simulink model "QBot2e_Image_Proc_Blob_Tracking"  (Simulink 8.9)
settings: Solver=ode1  StartTime=0.0  StopTime=inf  FixedStep=0.01  RelTol=1e-3  EnableMultiTasking=on
undefined symbols (not defined in the file): gcbh, HIL, JPEG, qc_get_step_size, Video3D, video_display_show
libraries: quarc_library x14
settings Model: Creator=drmadill  LastModifiedBy=User  SimulationMode=external  ExtModeTrigDuration=2
settings SolverCC: PositivePriorityOrder=on
settings OptimizationCC: ExpressionDepthLimit=2147483647  LifeSpan=auto
settings DebuggingCC: SolverPrmCheckMsg=warning
settings RTWCC: SystemTargetFile=quarc_linux_pi_3.tlc  TemplateMakefile=quarc_linux_pi_3_tmf  Description=QUARC Linux Raspberry Pi 3 Target
settings STFCustomTargetCC: TargetLibSuffix=.a  TargetPreCompLibLocation=C:\PROGRA~3\QUARC\lib\2019b\LINUX_~1\release  ConcurrentExecutionCompliant=on  SystemTargetFile=quarc_linux_pi_3.tlc
settings GRTTargetCC: TargetLibSuffix=.a  TargetPreCompLibLocation=C:\PROGRA~3\QUARC\lib\2017a\LICFC8~1\release  ParMdlRefBuildCompliant=off  CompOptLevelCompliant=off  GeneratePreprocessorConditionals=Use local settings  MatFileLogging=off  CPPClassGenCompliant=off  UseToolchainInfoCompliant=off  ExtMode=on  ExtModeMexFile=quarc_comm  ExtModeMexArgs='-w -d /tmp -uri %u'
settings ConfigComp: CovSFcnEnable=off

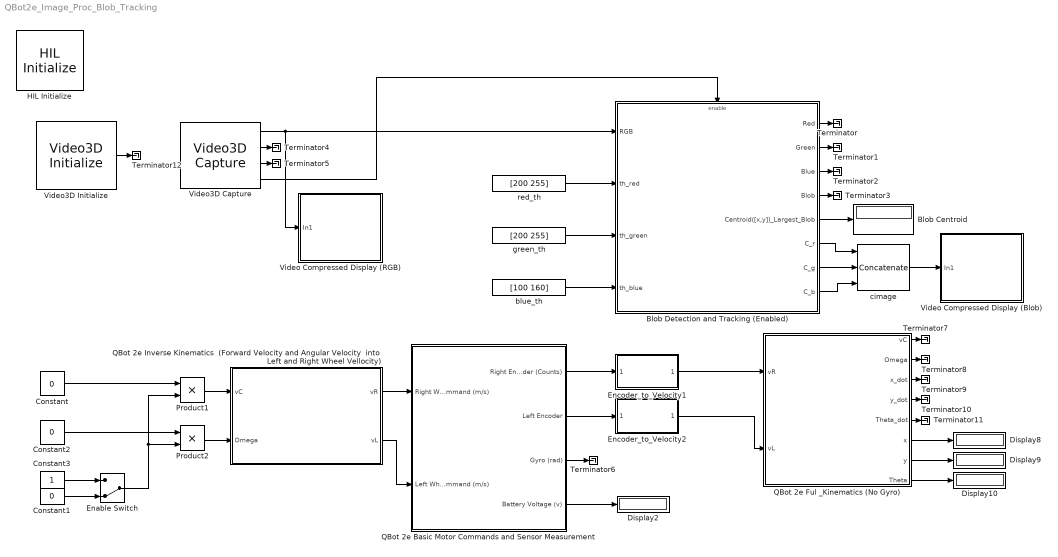
== system QBot2e_Image_Proc_Blob_Tracking ==
  " Blob Detection and Tracking (Enabled)" : Subsystem  TreatAsAtomicUnit=on
  Blob Centroid : Display
  Constant : Constant  Value=0
  Constant1 : Constant  Value=0
  Constant2 : Constant  Value=0
  Constant3 : Constant
  Display{2,8..10} (4 alike) : Display
  Enable Switch : ManualSwitch  CurrentSetting=0
  Encoder_to_Velocity1 : Subsystem
  Encoder_to_Velocity2 : Subsystem
  HIL Initialize : quarc_library/Data Acquisition/Generic/Configuration/HIL Initialize  Priority=-99  object_name=HIL-1  board_type=qbot2e  board_number=0  board_options=pwm0_en=1;pwm0_pin=12;pwm1_en=1;pwm1_pin=13;  exclusive=off  active=off  hardware_clocks=[]  clock_modes=[]  initial_clock_frequencies=[]  set_clock_params_at_start=off  set_clock_params_at_switch_in=off  set_clock_frequencies_at_start=off  set_clock_frequencies_at_switch_in=off  analog_input_channels=[0:5]  analog_input_configurations=[]  analog_input_maximums=[16.5 3.3 3.3 3.3 3.3 3.3]  analog_input_minimums=[0 0 0 0 0 0]  set_analog_input_params_at_start=off  set_analog_input_params_at_switch_in=off  analog_output_channels=[]  analog_output_maximums=[]  analog_output_minimums=[]  initial_analog_outputs=[]  final_analog_outputs=[]  watchdog_analog_outputs=[]  set_analog_output_params_at_start=off  set_analog_output_params_at_switch_in=off  set_analog_outputs_at_start=off  set_analog_outputs_at_switch_in=off  set_analog_outputs_at_terminate=off  set_analog_outputs_at_switch_out=off  set_analog_outputs_on_watchdog=off  digital_input_channels=[28:58]  digital_output_channels=[28:31]  digital_output_configuration=[]  initial_digital_outputs=[0]  final_digital_outputs=[0]  watchdog_digital_outputs=[]  set_digital_output_params_at_start=off  set_digital_output_params_at_switch_in=off  set_digital_outputs_at_start=on  set_digital_outputs_at_switch_in=off  set_digital_outputs_at_terminate=on  set_digital_outputs_at_switch_out=off  set_digital_outputs_on_watchdog=off  encoder_channels=[0:1]  quadrature=[4]  encoder_filter_frequency=[]  initial_encoder_counts=[0]  set_encoder_params_at_start=on  set_encoder_params_at_switch_in=off  set_encoder_counts_at_start=on  set_encoder_counts_at_switch_in=off  pwm_channels=[0:1]  pwm_modes=0  pwm_frequency=100e6 / 4095  pwm_configuration=[0]  pwm_alignment=[0]  pwm_polarity=[1]  pwm_leading_deadband=[]  pwm_trailing_deadband=[]  initial_pwm_outputs=[0]  final_pwm_outputs=[0]  watchdog_pwm_outputs=[]  set_pwm_params_at_start=on  set_pwm_params_at_switch_in=off  set_pwm_outputs_at_start=on  set_pwm_outputs_at_switch_in=off  set_pwm_outputs_at_terminate=on  set_pwm_outputs_at_switch_out=off  set_pwm_outputs_on_watchdog=off  other_output_channels=[2000:2001 14000 16000]  initial_other_outputs=[0 0 0 7]  final_other_outputs=[0 0 0 7]  watchdog_other_outputs=[]  set_other_outputs_at_start=on  set_other_outputs_at_switch_in=off  set_other_outputs_at_terminate=on  set_other_outputs_at_switch_out=off  set_other_outputs_on_watchdog=off
  Product1 : Product  RndMeth=Zero
  Product2 : Product  RndMeth=Zero
  QBot 2e Basic Motor Commands and Sensor Measurement : Subsystem
  QBot 2e Ful _Kinematics (No Gyro) : Subsystem
  QBot 2e Inverse Kinematics  (Forward Velocity and Angular Velocity  into Left and Right Wheel Vellocity) : Subsystem
  Terminator{,1..12} (13 alike) : Terminator
  Video Compressed Display (Blob) : Subsystem  LoadFcn=set_param(gcbh, 'UserData', gcb);  StartFcn=video_display_show([gcb, '/Video Display'], 'add', gcb);  mask(Video Compressed Display){algorithm=JPEG, quality=50, sample_time=-1, use_hardware=on}
      mask prompts: algorithm "Compression algorithm:"; quality "Compression quality (0-100):"; sample_time "Sample time (seconds):"; use_hardware "Use hardware acceleration for video display"
      mask help: Displays a video stream on the host, using compression to minimize bandwidth.
      mask init:
      | qc_set_display('Video\nCompressed\nDisplay');
      settings: UndoDeleteFcn=set_param(gcbh, 'UserData', gcb);  OpenFcn=video_display_show([gcb, '/Video Display'], 'show', gcb);  PreDeleteFcn=video_display_show([gcb, '/Video Display'], 'delete');
      settings: CopyFcn=|
      | set_param(gcbh, 'UserData', gcb);
      | set_param(gcbh, 'LinkStatus', 'none');
      settings: NameChangeFcn=|
      | video_display_show([get_param(gcbh, 'UserData'), '/Video Display'], 'rename', [gcb, '/Video Display']);
      | video_display_show([gcb, '/Video Display'], 'add', gcb);
      | set_param(gcbh, 'UserData', gcb);
      mask Help: web(qc_get_block_help_path(gcb));
      mask TypeOptions algorithm: Image Compress/algorithm
      mask TypeOptions quality: Image Compress/quality
      mask TypeOptions sample_time: Video Display/sample_time
      mask TypeOptions use_hardware: Video Display/use_hardware
      mask Display:
      | patch([0.98591 0.98591 0.62618 0.59072 0.56147   0.536   0.536  0.5441 0.56912 0.59207 0.60881 0.62276 0.63527 0.64364  0.6485  0.6485 0.64706 0.64499 0.63662 0.62411 0.61232 0.59837 0.58307 0.56147   0.536   0.536  0.5441  0.5747 0.60953 0.63662 0.67001  0.7034 0.72851 0.75425 0.77927 0.80294 0.82454 0.84119 0.85865 0.87395 0.88574 0.89339  0.8969 0.89969 0.89969 0.89267  0.8816 0.87044 0.85649  0.8384 0.81824 0.80294 0.78764 0.77513 0.76676 0.75776 0.76397 0.77513 0.79178 0.80987 0.82796 0.84326 0.86207 0.98528],[0.18689 0.05522 0.05522 0.05171 0.05171    0.05 0.18338 0.18338 0.19148 0.20435 0.22298 0.24863 0.28589 0.33125 0.38138 0.55139 0.59801 0.63761 0.68189 0.72149 0.74939 0.76694 0.77855 0.79367 0.79952 0.92768 0.92768 0.92768 0.92417 0.92066 0.91364  0.9032 0.89384 0.88106 0.86594 0.85073 0.82634 0.80537 0.77855 0.74363 0.70403 0.65858 0.61079 0.59099 0.41513 0.37202 0.31847 0.29048 0.25556 0.23342  0.2102 0.19382 0.18221 0.17285 0.16943 0.16124  0.1589 0.16241 0.16709 0.17168  0.1787 0.18221 0.18689 0.18689],[0.9,0.90,0.91])
      | patch([0.536 0.52601 0.46823 0.44528 0.41603 0.39101 0.35555 0.33116 0.31451 0.29291  0.2804 0.26717 0.25322 0.23999 0.22406 0.20732 0.19337 0.17528 0.15935 0.14396 0.13217 0.11759 0.10922 0.10085 0.09671 0.09392 0.09041 0.08906 0.08906 0.09464  0.0995 0.10778 0.11894 0.13145 0.14675 0.16349 0.17672 0.19409 0.20732 0.22406 0.23999 0.26159 0.27833 0.29849 0.31793 0.33602 0.35411 0.37085 0.39245 0.41603   0.536   0.536 0.53159 0.46409   0.446 0.42026 0.39587 0.37571 0.36113 0.34925 0.34088 0.33809 0.33809 0.34088 0.34583 0.35627 0.36392 0.38129 0.39587 0.41117 0.42719 0.44672  0.4676 0.48353 0.48353 0.52394   0.536],[0.05 0.04829 0.04712 0.04712 0.04829 0.05063 0.05405 0.05873 0.06107 0.06692 0.07043 0.07619 0.08087 0.08672 0.09482 0.10652 0.11696 0.13325  0.1508 0.17168 0.19499 0.22415 0.25439 0.28472 0.31379 0.35456 0.38489 0.41513 0.58055 0.63878 0.68774 0.72149 0.75641 0.78089 0.80537 0.82859 0.84029 0.85658 0.86594 0.87404  0.8834 0.89267 0.90086 0.90788 0.91247 0.91832 0.92066   0.923 0.92651 0.92768 0.92768 0.79952 0.79952 0.79952 0.79718 0.78899 0.77153 0.75056 0.72149 0.68072 0.62249  0.5549 0.41396 0.37085 0.33242 0.28121 0.25205 0.22181 0.20552 0.19499 0.18572 0.18221 0.17753 0.17636 0.17753  0.1787  0.1787],[0.9,0.90,0.91])
      | disp('Video\nCompressed\nDisplay');
  Video Compressed Display (RGB) : Subsystem  LoadFcn=set_param(gcbh, 'UserData', gcb);  StartFcn=video_display_show([gcb, '/Video Display'], 'add', gcb);  mask(Video Compressed Display){algorithm=JPEG, quality=50, sample_time=-1, use_hardware=on}
      mask prompts: algorithm "Compression algorithm:"; quality "Compression quality (0-100):"; sample_time "Sample time (seconds):"; use_hardware "Use hardware acceleration for video display"
      mask help: Displays a video stream on the host, using compression to minimize bandwidth.
      mask init:
      | qc_set_display('Video\nCompressed\nDisplay');
      settings: UndoDeleteFcn=set_param(gcbh, 'UserData', gcb);  OpenFcn=video_display_show([gcb, '/Video Display'], 'show', gcb);  PreDeleteFcn=video_display_show([gcb, '/Video Display'], 'delete');
      settings: CopyFcn=|
      | set_param(gcbh, 'UserData', gcb);
      | set_param(gcbh, 'LinkStatus', 'none');
      settings: NameChangeFcn=|
      | video_display_show([get_param(gcbh, 'UserData'), '/Video Display'], 'rename', [gcb, '/Video Display']);
      | video_display_show([gcb, '/Video Display'], 'add', gcb);
      | set_param(gcbh, 'UserData', gcb);
      mask Help: web(qc_get_block_help_path(gcb));
      mask TypeOptions algorithm: Image Compress/algorithm
      mask TypeOptions quality: Image Compress/quality
      mask TypeOptions sample_time: Video Display/sample_time
      mask TypeOptions use_hardware: Video Display/use_hardware
      mask Display:
      | patch([0.98591 0.98591 0.62618 0.59072 0.56147   0.536   0.536  0.5441 0.56912 0.59207 0.60881 0.62276 0.63527 0.64364  0.6485  0.6485 0.64706 0.64499 0.63662 0.62411 0.61232 0.59837 0.58307 0.56147   0.536   0.536  0.5441  0.5747 0.60953 0.63662 0.67001  0.7034 0.72851 0.75425 0.77927 0.80294 0.82454 0.84119 0.85865 0.87395 0.88574 0.89339  0.8969 0.89969 0.89969 0.89267  0.8816 0.87044 0.85649  0.8384 0.81824 0.80294 0.78764 0.77513 0.76676 0.75776 0.76397 0.77513 0.79178 0.80987 0.82796 0.84326 0.86207 0.98528],[0.18689 0.05522 0.05522 0.05171 0.05171    0.05 0.18338 0.18338 0.19148 0.20435 0.22298 0.24863 0.28589 0.33125 0.38138 0.55139 0.59801 0.63761 0.68189 0.72149 0.74939 0.76694 0.77855 0.79367 0.79952 0.92768 0.92768 0.92768 0.92417 0.92066 0.91364  0.9032 0.89384 0.88106 0.86594 0.85073 0.82634 0.80537 0.77855 0.74363 0.70403 0.65858 0.61079 0.59099 0.41513 0.37202 0.31847 0.29048 0.25556 0.23342  0.2102 0.19382 0.18221 0.17285 0.16943 0.16124  0.1589 0.16241 0.16709 0.17168  0.1787 0.18221 0.18689 0.18689],[0.9,0.90,0.91])
      | patch([0.536 0.52601 0.46823 0.44528 0.41603 0.39101 0.35555 0.33116 0.31451 0.29291  0.2804 0.26717 0.25322 0.23999 0.22406 0.20732 0.19337 0.17528 0.15935 0.14396 0.13217 0.11759 0.10922 0.10085 0.09671 0.09392 0.09041 0.08906 0.08906 0.09464  0.0995 0.10778 0.11894 0.13145 0.14675 0.16349 0.17672 0.19409 0.20732 0.22406 0.23999 0.26159 0.27833 0.29849 0.31793 0.33602 0.35411 0.37085 0.39245 0.41603   0.536   0.536 0.53159 0.46409   0.446 0.42026 0.39587 0.37571 0.36113 0.34925 0.34088 0.33809 0.33809 0.34088 0.34583 0.35627 0.36392 0.38129 0.39587 0.41117 0.42719 0.44672  0.4676 0.48353 0.48353 0.52394   0.536],[0.05 0.04829 0.04712 0.04712 0.04829 0.05063 0.05405 0.05873 0.06107 0.06692 0.07043 0.07619 0.08087 0.08672 0.09482 0.10652 0.11696 0.13325  0.1508 0.17168 0.19499 0.22415 0.25439 0.28472 0.31379 0.35456 0.38489 0.41513 0.58055 0.63878 0.68774 0.72149 0.75641 0.78089 0.80537 0.82859 0.84029 0.85658 0.86594 0.87404  0.8834 0.89267 0.90086 0.90788 0.91247 0.91832 0.92066   0.923 0.92651 0.92768 0.92768 0.79952 0.79952 0.79952 0.79718 0.78899 0.77153 0.75056 0.72149 0.68072 0.62249  0.5549 0.41396 0.37085 0.33242 0.28121 0.25205 0.22181 0.20552 0.19499 0.18572 0.18221 0.17753 0.17636 0.17753  0.1787  0.1787],[0.9,0.90,0.91])
      | disp('Video\nCompressed\nDisplay');
  Video3D Capture : quarc_library/Multimedia/Video3D Capture  object_name=Video3D-1  stream_type=RGB  stream_index=0  resolution=640 x 480  width=640  height=480  output_format=MATLAB RGB (HxWx3)  data_type=uint8  sample_time=qc_get_step_size * ceil(0.033 / qc_get_step_size)  brightness_override=off  brightness=50.0  contrast_override=off  contrast=50.0  hue_override=off  hue=50.0  saturation_override=off  saturation=50.0  sharpness_override=off  sharpness=50.0  gamma_override=off  gamma=50.0  gain_override=off  gain=50.0  backlightcompensation_override=off  backlightcompensation=50.0  whitebalance_override=Automatic white balance  whitebalance=50.0  exposure_override=Automatic exposure  exposure=30.0  emitter=Enable laser emitter  preset=Do not set camera presets
  Video3D Initialize : quarc_library/Multimedia/Video3D Initialize  object_name=Video3D-1  source=Device  identifier=0  file=sample.bag  sample_time=qc_get_step_size * ceil(0.033 / qc_get_step_size)  active=on
  blue_th : Constant  Value=[100 160]
  cimage : Concatenate  NumInputs=3  Mode=Multidimensional array  ConcatenateDimension=3
  green_th : Constant  Value=[200 255]
  red_th : Constant  Value=[200 255]
  wires:
  red_th/1 -> " Blob Detection and Tracking (Enabled)"/2(th_red)
  green_th/1 -> " Blob Detection and Tracking (Enabled)"/3(th_green)
  blue_th/1 -> " Blob Detection and Tracking (Enabled)"/4(th_blue)
  " Blob Detection and Tracking (Enabled)"/5(Centroid([x,y])_Largest_Blob) -> Blob Centroid/1
  " Blob Detection and Tracking (Enabled)"/6(C_r) -> cimage/1
  " Blob Detection and Tracking (Enabled)"/7(C_g) -> cimage/2
  " Blob Detection and Tracking (Enabled)"/8(C_b) -> cimage/3
  Constant3/1 -> Enable Switch/1
  Constant1/1 -> Enable Switch/2
  QBot 2e Basic Motor Commands and Sensor Measurement/1(Right Encoder (Counts)) -> Encoder_to_Velocity1/1(Encoder)
  QBot 2e Ful _Kinematics (No Gyro)/8(Theta) -> Display10/1
  QBot 2e Ful _Kinematics (No Gyro)/7(y) -> Display9/1
  QBot 2e Ful _Kinematics (No Gyro)/6(x) -> Display8/1
  Encoder_to_Velocity1/1(Velocity) -> QBot 2e Ful _Kinematics (No Gyro)/1(vR)
  Encoder_to_Velocity2/1(Velocity) -> QBot 2e Ful _Kinematics (No Gyro)/2(vL)
  Constant/1 -> Product1/1
  Constant2/1 -> Product2/1
  QBot 2e Inverse Kinematics  (Forward Velocity and Angular Velocity  into Left and Right Wheel Vellocity)/1(vR) -> QBot 2e Basic Motor Commands and Sensor Measurement/1(Right Wheel Command (m/s))
  QBot 2e Inverse Kinematics  (Forward Velocity and Angular Velocity  into Left and Right Wheel Vellocity)/2(vL) -> QBot 2e Basic Motor Commands and Sensor Measurement/2(Left Wheel Command (m/s))
  Product1/1 -> QBot 2e Inverse Kinematics  (Forward Velocity and Angular Velocity  into Left and Right Wheel Vellocity)/1(vC)
  Product2/1 -> QBot 2e Inverse Kinematics  (Forward Velocity and Angular Velocity  into Left and Right Wheel Vellocity)/2(Omega)
  Enable Switch/1 -> Product1/2, Product2/2
  " Blob Detection and Tracking (Enabled)"/1(Red) -> Terminator/1
  " Blob Detection and Tracking (Enabled)"/2(Green) -> Terminator1/1
  " Blob Detection and Tracking (Enabled)"/3(Blue) -> Terminator2/1
  " Blob Detection and Tracking (Enabled)"/4(Blob) -> Terminator3/1
  QBot 2e Ful _Kinematics (No Gyro)/1(vC) -> Terminator7/1
  QBot 2e Ful _Kinematics (No Gyro)/2(Omega) -> Terminator8/1
  QBot 2e Ful _Kinematics (No Gyro)/3(x_dot) -> Terminator9/1
  QBot 2e Ful _Kinematics (No Gyro)/4(y_dot) -> Terminator10/1
  QBot 2e Ful _Kinematics (No Gyro)/5(Theta_dot) -> Terminator11/1
  cimage/1 -> Video Compressed Display (Blob)/1(In1)
  QBot 2e Basic Motor Commands and Sensor Measurement/2(Left Encoder) -> Encoder_to_Velocity2/1(Encoder)
  QBot 2e Basic Motor Commands and Sensor Measurement/4(Battery Voltage (v)) -> Display2/1
  QBot 2e Basic Motor Commands and Sensor Measurement/3(Gyro (rad)) -> Terminator6/1
  Video3D Initialize/1 -> Terminator12/1
  Video3D Capture/4 -> " Blob Detection and Tracking (Enabled)"/Enable
  Video3D Capture/1 -> Video Compressed Display (RGB)/1(In1), " Blob Detection and Tracking (Enabled)"/1(RGB)
  Video3D Capture/2 -> Terminator4/1
  Video3D Capture/3 -> Terminator5/1

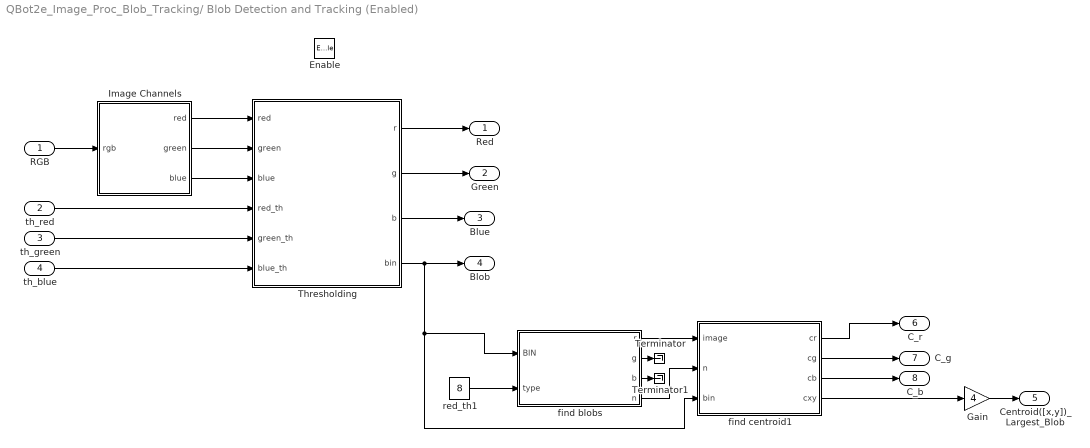
== system QBot2e_Image_Proc_Blob_Tracking/ Blob Detection and Tracking (Enabled) ==
  RGB : Inport
  th_red : Inport  Port=2
  th_green : Inport  Port=3
  th_blue : Inport  Port=4
  Enable : EnablePort
  Gain : Gain  Gain=4
  Image Channels : Subsystem
  Terminator : Terminator
  Terminator1 : Terminator
  Thresholding : MATLAB Function  TreatAsAtomicUnit=on
  find blobs : MATLAB Function  TreatAsAtomicUnit=on
  find centroid1 : MATLAB Function  TreatAsAtomicUnit=on
  red_th1 : Constant  Value=8
  Red : Outport
  Green : Outport  Port=2
  Blue : Outport  Port=3
  Blob : Outport  Port=4
  Centroid([x,y])_Largest_Blob : Outport  Port=5
  C_r : Outport  Port=6
  C_g : Outport  Port=7
  C_b : Outport  Port=8
  wires:
  th_red/1 -> Thresholding/4(red_th)
  th_green/1 -> Thresholding/5(green_th)
  th_blue/1 -> Thresholding/6(blue_th)
  Thresholding/1(r) -> Red/1
  Thresholding/2(g) -> Green/1
  Thresholding/3(b) -> Blue/1
  red_th1/1 -> find blobs/2(type)
  find blobs/1(r) -> find centroid1/1(image)
  find blobs/4(n) -> find centroid1/2(n)
  Gain/1 -> Centroid([x,y])_Largest_Blob/1
  Thresholding/4(bin) -> Blob/1, find blobs/1(BIN), find centroid1/3(bin)
  find centroid1/4(cxy) -> Gain/1
  find centroid1/1(cr) -> C_r/1
  find centroid1/2(cg) -> C_g/1
  find centroid1/3(cb) -> C_b/1
  Image Channels/1(red) -> Thresholding/1(red)
  Image Channels/2(green) -> Thresholding/2(green)
  Image Channels/3(blue) -> Thresholding/3(blue)
  RGB/1 -> Image Channels/1(rgb)
  find blobs/2(g) -> Terminator/1
  find blobs/3(b) -> Terminator1/1

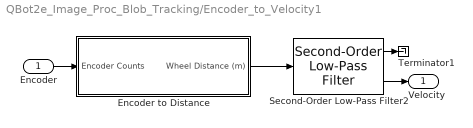
== system QBot2e_Image_Proc_Blob_Tracking/Encoder_to_Velocity1 ==
  Encoder : Inport
  Encoder to Distance : Subsystem
  Second-Order Low-Pass Filter2 : quarc_library/Continuous/Second-Order Low-Pass Filter  params_source=Internal (dialog parameters)  input_width=10  input_zeta=1  input_init=0
  Terminator1 : Terminator
  Velocity : Outport
  wires:
  Second-Order Low-Pass Filter2/1 -> Terminator1/1
  Encoder to Distance/1(Wheel Distance (m)) -> Second-Order Low-Pass Filter2/1
  Encoder/1 -> Encoder to Distance/1(Encoder Counts)
  Second-Order Low-Pass Filter2/2 -> Velocity/1

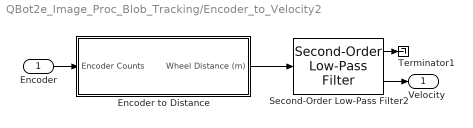
== system QBot2e_Image_Proc_Blob_Tracking/Encoder_to_Velocity2 ==
  Encoder : Inport
  Encoder to Distance : Subsystem
  Second-Order Low-Pass Filter2 : quarc_library/Continuous/Second-Order Low-Pass Filter  params_source=Internal (dialog parameters)  input_width=10  input_zeta=1  input_init=0
  Terminator1 : Terminator
  Velocity : Outport
  wires:
  Second-Order Low-Pass Filter2/2 -> Velocity/1
  Encoder/1 -> Encoder to Distance/1(Encoder Counts)
  Encoder to Distance/1(Wheel Distance (m)) -> Second-Order Low-Pass Filter2/1
  Second-Order Low-Pass Filter2/1 -> Terminator1/1

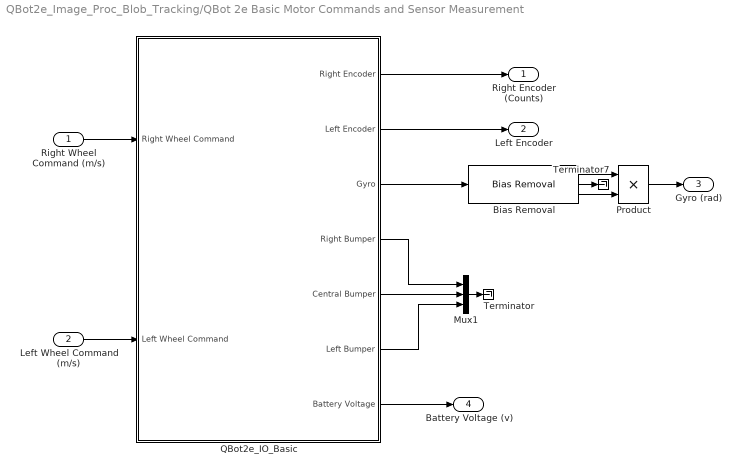
== system QBot2e_Image_Proc_Blob_Tracking/QBot 2e Basic Motor Commands and Sensor Measurement ==
  Right Wheel Command (m/s) : Inport
  Left Wheel Command (m/s) : Inport  Port=2
  Bias Removal : quarc_library/Discrete/Bias Removal  start_time=3  end_time=4  switch_id=0  sample_time=qc_get_step_size
      settings: SourceProductName=QUARC Targets
  Mux1 : Mux  Inputs=3
  Product : Product  RndMeth=Zero
  QBot2e_IO_Basic : Subsystem
  Terminator : Terminator
  Terminator7 : Terminator
  Right Encoder (Counts) : Outport
  Left Encoder : Outport  Port=2
  Gyro (rad) : Outport  Port=3
  Battery Voltage (v) : Outport  Port=4
  wires:
  QBot2e_IO_Basic/4(Right Bumper) -> Mux1/1
  QBot2e_IO_Basic/5(Central Bumper) -> Mux1/2
  QBot2e_IO_Basic/6(Left Bumper) -> Mux1/3
  Right Wheel Command (m/s)/1 -> QBot2e_IO_Basic/1(Right Wheel Command)
  Left Wheel Command (m/s)/1 -> QBot2e_IO_Basic/2(Left Wheel Command)
  QBot2e_IO_Basic/1(Right Encoder) -> Right Encoder (Counts)/1
  QBot2e_IO_Basic/2(Left Encoder) -> Left Encoder/1
  QBot2e_IO_Basic/7(Battery Voltage) -> Battery Voltage (v)/1
  Bias Removal/2 -> Terminator7/1
  Bias Removal/1 -> Product/1
  Bias Removal/3 -> Product/2
  Product/1 -> Gyro (rad)/1
  QBot2e_IO_Basic/3(Gyro) -> Bias Removal/1
  Mux1/1 -> Terminator/1

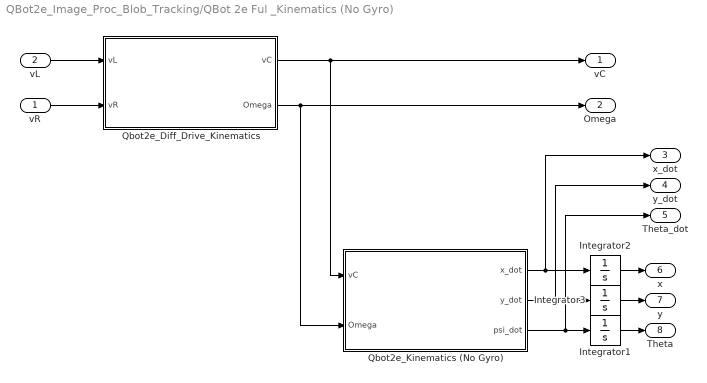
== system QBot2e_Image_Proc_Blob_Tracking/QBot 2e Ful _Kinematics (No Gyro) ==
  vR : Inport
  vL : Inport  Port=2
  Integrator1 : Integrator
  Integrator2 : Integrator
  Integrator3 : Integrator
  Qbot2e_Diff_Drive_Kinematics : Subsystem
  Qbot2e_Kinematics (No Gyro) : Subsystem
  vC : Outport
  Omega : Outport  Port=2
  x_dot : Outport  Port=3
  y_dot : Outport  Port=4
  Theta_dot : Outport  Port=5
  x : Outport  Port=6
  y : Outport  Port=7
  Theta : Outport  Port=8
  wires:
  Integrator1/1 -> Theta/1
  Qbot2e_Kinematics (No Gyro)/3(psi_dot) -> Theta_dot/1, Integrator1/1
  Qbot2e_Kinematics (No Gyro)/1(x_dot) -> x_dot/1, Integrator2/1
  Qbot2e_Kinematics (No Gyro)/2(y_dot) -> y_dot/1, Integrator3/1
  Qbot2e_Diff_Drive_Kinematics/1(vC) -> Qbot2e_Kinematics (No Gyro)/1(vC), vC/1
  vL/1 -> Qbot2e_Diff_Drive_Kinematics/1(vL)
  vR/1 -> Qbot2e_Diff_Drive_Kinematics/2(vR)
  Integrator2/1 -> x/1
  Integrator3/1 -> y/1
  Qbot2e_Diff_Drive_Kinematics/2(Omega) -> Qbot2e_Kinematics (No Gyro)/2(Omega), Omega/1

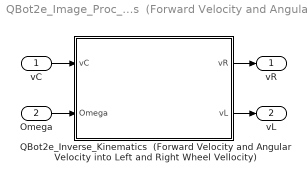
== system QBot2e_Image_Proc_Blob_Tracking/QBot 2e Inverse Kinematics  (Forward Velocity and Angular Velocity  into Left and Right Wheel Vellocity) ==
  vC : Inport
  Omega : Inport  Port=2
  QBot2e_Inverse_Kinematics  (Forward Velocity and Angular Velocity into Left and Right Wheel Vellocity) : MATLAB Function  TreatAsAtomicUnit=on
  vR : Outport
  vL : Outport  Port=2
  wires:
  QBot2e_Inverse_Kinematics  (Forward Velocity and Angular Velocity into Left and Right Wheel Vellocity)/2(vL) -> vL/1
  Omega/1 -> QBot2e_Inverse_Kinematics  (Forward Velocity and Angular Velocity into Left and Right Wheel Vellocity)/2(Omega)
  QBot2e_Inverse_Kinematics  (Forward Velocity and Angular Velocity into Left and Right Wheel Vellocity)/1(vR) -> vR/1
  vC/1 -> QBot2e_Inverse_Kinematics  (Forward Velocity and Angular Velocity into Left and Right Wheel Vellocity)/1(vC)

== system QBot2e_Image_Proc_Blob_Tracking/Video Compressed Display (Blob) ==
  In1 : Inport
  Channel : quarc_library/Signal Routing/Channel  channel=0  buffer_size=1
  Image Compress : quarc_library/Image Processing/Generic/Image Compress  algorithm=JPEG  source=Internal dialog parameter  quality=quality  output_dim=-1
  Video Display : quarc_library/Multimedia/Video Display  Tag=|  sample_time=sample_time  use_hardware=on
      | QBot2e_Image_Proc_Blob_Tracking/Video Compressed
      | Display (Blob)/Video Display
  wires:
  Channel/1 -> Video Display/1
  In1/1 -> Image Compress/1
  Image Compress/1 -> Channel/1

== system QBot2e_Image_Proc_Blob_Tracking/Video Compressed Display (RGB) ==
  In1 : Inport
  Channel : quarc_library/Signal Routing/Channel  channel=1  buffer_size=1
  Image Compress : quarc_library/Image Processing/Generic/Image Compress  algorithm=JPEG  source=Internal dialog parameter  quality=quality  output_dim=-1
  Video Display : quarc_library/Multimedia/Video Display  Tag=|  sample_time=sample_time  use_hardware=on
      | QBot2e_Image_Proc_Blob_Tracking/Video Compressed
      | Display (RGB)/Video Display
  wires:
  Image Compress/1 -> Channel/1
  In1/1 -> Image Compress/1
  Channel/1 -> Video Display/1

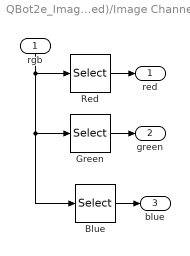
== system QBot2e_Image_Proc_Blob_Tracking/ Blob Detection and Tracking (Enabled)/Image Channels ==
  rgb : Inport
  Blue : Selector  NumberOfDimensions=3  InputPortWidth=3  IndexOptions=Select all,Select all,Index vector (dialog)  Indices=1,1,3  OutputSizes=1,1,1
  Green : Selector  NumberOfDimensions=3  InputPortWidth=3  IndexOptions=Select all,Select all,Index vector (dialog)  Indices=1,1,2  OutputSizes=1,1,1
  Red : Selector  NumberOfDimensions=3  InputPortWidth=3  IndexOptions=Select all,Select all,Index vector (dialog)  Indices=[1 3],1,1  OutputSizes=1,1,1
  red : Outport
  green : Outport  Port=2
  blue : Outport  Port=3
  wires:
  rgb/1 -> Red/1, Blue/1, Green/1
  Red/1 -> red/1
  Green/1 -> green/1
  Blue/1 -> blue/1

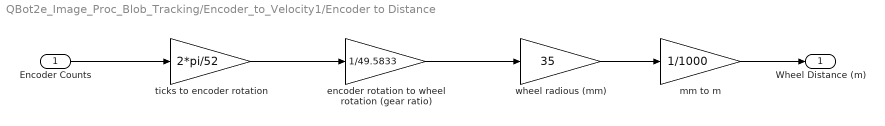
== system QBot2e_Image_Proc_Blob_Tracking/Encoder_to_Velocity1/Encoder to Distance ==
  Encoder Counts : Inport
  " encoder rotation to wheel rotation (gear ratio)" : Gain  Gain=1/49.5833
  mm to m : Gain  Gain=1/1000
  ticks to encoder rotation : Gain  Gain=2*pi/52
  wheel radious (mm) : Gain  Gain=35
  Wheel Distance (m) : Outport
  wires:
  Encoder Counts/1 -> ticks to encoder rotation/1
  ticks to encoder rotation/1 -> " encoder rotation to wheel rotation (gear ratio)"/1
  " encoder rotation to wheel rotation (gear ratio)"/1 -> wheel radious (mm)/1
  wheel radious (mm)/1 -> mm to m/1
  mm to m/1 -> Wheel Distance (m)/1

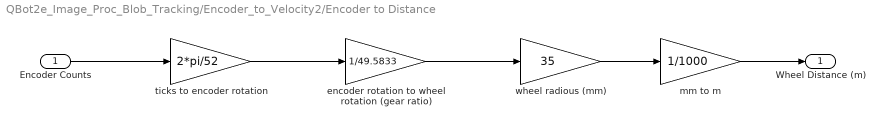
== system QBot2e_Image_Proc_Blob_Tracking/Encoder_to_Velocity2/Encoder to Distance ==
  Encoder Counts : Inport
  " encoder rotation to wheel rotation (gear ratio)" : Gain  Gain=1/49.5833
  mm to m : Gain  Gain=1/1000
  ticks to encoder rotation : Gain  Gain=2*pi/52
  wheel radious (mm) : Gain  Gain=35
  Wheel Distance (m) : Outport
  wires:
  mm to m/1 -> Wheel Distance (m)/1
  wheel radious (mm)/1 -> mm to m/1
  " encoder rotation to wheel rotation (gear ratio)"/1 -> wheel radious (mm)/1
  ticks to encoder rotation/1 -> " encoder rotation to wheel rotation (gear ratio)"/1
  Encoder Counts/1 -> ticks to encoder rotation/1

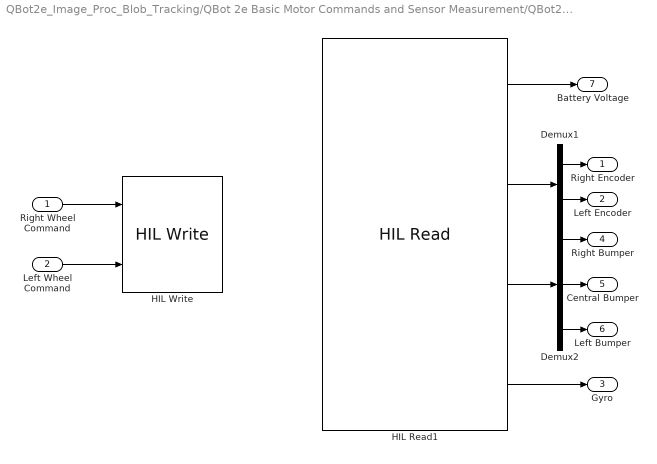
== system QBot2e_Image_Proc_Blob_Tracking/QBot 2e Basic Motor Commands and Sensor Measurement/QBot2e_IO_Basic ==
  Right Wheel Command : Inport
  Left Wheel Command : Inport  Port=2
  Demux1 : Demux  Outputs=2
  Demux2 : Demux  Outputs=3
  HIL Read1 : quarc_library/Data Acquisition/Generic/Immediate I//O/HIL Read  object_name=HIL-1  analog_channels=[0]  encoder_channels=[0:1]  digital_channels=[28:30]  other_channels=[1002]  sample_time=qc_get_step_size  active=on  vector_output=on  data_type_mode=Inherit via back propagation  encoder_data_type=double  digital_data_type=boolean
  HIL Write : quarc_library/Data Acquisition/Generic/Immediate I//O/HIL Write  object_name=HIL-1  analog_channels=[]  pwm_channels=[]  digital_channels=[]  other_channels=[2000:2001]  sample_time=-1  active=on  vector_input=off
  Right Encoder : Outport
  Left Encoder : Outport  Port=2
  Gyro : Outport  Port=3
  Right Bumper : Outport  Port=4
  Central Bumper : Outport  Port=5
  Left Bumper : Outport  Port=6
  Battery Voltage : Outport  Port=7
  wires:
  HIL Read1/1 -> Battery Voltage/1
  HIL Read1/3 -> Demux2/1
  HIL Read1/4 -> Gyro/1
  Demux1/1 -> Right Encoder/1
  Demux1/2 -> Left Encoder/1
  Right Wheel Command/1 -> HIL Write/1
  Left Wheel Command/1 -> HIL Write/2
  HIL Read1/2 -> Demux1/1
  Demux2/1 -> Right Bumper/1
  Demux2/2 -> Central Bumper/1
  Demux2/3 -> Left Bumper/1

== system QBot2e_Image_Proc_Blob_Tracking/QBot 2e Ful _Kinematics (No Gyro)/Qbot2e_Diff_Drive_Kinematics ==
  vL : Inport
  vR : Inport  Port=2
  Qbot2_Diff_Drive_Kinematics : MATLAB Function  TreatAsAtomicUnit=on
  vC : Outport
  Omega : Outport  Port=2
  wires:
  vL/1 -> Qbot2_Diff_Drive_Kinematics/1(vL)
  Qbot2_Diff_Drive_Kinematics/1(vC) -> vC/1
  vR/1 -> Qbot2_Diff_Drive_Kinematics/2(vR)
  Qbot2_Diff_Drive_Kinematics/2(Omega) -> Omega/1

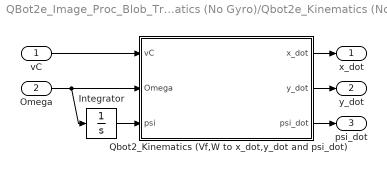
== system QBot2e_Image_Proc_Blob_Tracking/QBot 2e Ful _Kinematics (No Gyro)/Qbot2e_Kinematics (No Gyro) ==
  vC : Inport
  Omega : Inport  Port=2
  Integrator : Integrator
  Qbot2_Kinematics (Vf,W to x_dot,y_dot and psi_dot) : MATLAB Function  TreatAsAtomicUnit=on
  x_dot : Outport
  y_dot : Outport  Port=2
  psi_dot : Outport  Port=3
  wires:
  Qbot2_Kinematics (Vf,W to x_dot,y_dot and psi_dot)/3(psi_dot) -> psi_dot/1
  Integrator/1 -> Qbot2_Kinematics (Vf,W to x_dot,y_dot and psi_dot)/3(psi)
  vC/1 -> Qbot2_Kinematics (Vf,W to x_dot,y_dot and psi_dot)/1(vC)
  Qbot2_Kinematics (Vf,W to x_dot,y_dot and psi_dot)/1(x_dot) -> x_dot/1
  Omega/1 -> Integrator/1, Qbot2_Kinematics (Vf,W to x_dot,y_dot and psi_dot)/2(Omega)
  Qbot2_Kinematics (Vf,W to x_dot,y_dot and psi_dot)/2(y_dot) -> y_dot/1

== matlab function  Blob Detection and Tracking (Enabled)/find centroid1 ==
  data: cr output double; cg output double; cb output double; image input double; cxy output double; n input double; bin input double
function [cr, cg, cb, cxy]  = find_centroid(image, n, bin)
% This block supports the Embedded MATLAB subset.
% See the help menu for details. 

[binrow bincol] = size(bin);
cr = bin;
cg = bin;
cb = bin;
[row col] = size(image);
x = -1;
y = -1;
cxy = zeros(2,1);
if n>50
    cxy(1,1) = x;
    cxy(2,1) = y;
    return;
end
X = zeros(1, 50);
Y = zeros(1, 50);
N = zeros(1, 50);
for L=1:n
    for i=1:row
        for j=1:col
            if image(i, j) == L
                X(L) = X(L) + j;
                Y(L) = Y(L) + i;
                N(L) = N(L) + 1;
            end
        end
    end
end

maxN = -1;
maxNid = -1;
for L=1:n
    val = N(L);
    if val > maxN
        maxN = val;
        maxNid = L;
    end
end

if maxN > 0
    x = 4*(X(maxNid)/N(maxNid));
    y = 4*(Y(maxNid)/N(maxNid));
    
    for i=fix(y-2):fix(y+2)
        if i>=1 && i<=binrow
            for j=fix(x-2):fix(x+2) 
                if j>=1 && j<=bincol
                    cr(i, j) = 255;
                    cg(i, j) = 0;
                    cb(i, j) = 0;
                end
            end
        end
    end
    
end

cxy(1,1) = x;
cxy(2,1) = y;

return;
%--------------------------------------------------------------------------

== matlab function QBot 2e Ful _Kinematics (No Gyro)/Qbot2e_Diff_Drive_Kinematics/Qbot2_Diff_Drive_Kinematics ==
  data: vL input double; vC output double; vR input double; Omega output double
function [vC,Omega] = fcn(vL,vR)
%#codegen

d= 0.235;

vC=0.5*(vL+vR);
Omega=(1/d)*(vR-vL);

== matlab function  Blob Detection and Tracking (Enabled)/Thresholding ==
  data: red input double; r output double; g output double; b output double; bin output double; green input double; blue input double; red_th input double; green_th input double; blue_th input double
function [r, g, b, bin]  = clr_thr(red, ...
    green, blue, red_th, green_th, blue_th)
% This block supports the Embedded MATLAB subset.
% See the help menu for details. 

red_vec = thresh(red, red_th, 1);

green_vec = thresh(green, green_th, 1);

blue_vec = thresh(blue, blue_th, 1);

tmp = double(and(red_vec, green_vec));
tmp_blob = uint8(and(tmp, blue_vec));
bin = uint8(255*tmp_blob);

% background = uint8(255*double(not(tmp_blob)));
% r = uint8(red.*tmp_blob + background);
% g = uint8(green.*tmp_blob + background);
% b = uint8(blue.*tmp_blob + background);

r = uint8(red.*tmp_blob);
g = uint8(green.*tmp_blob);
b = uint8(blue.*tmp_blob);


return;

%--------------------------------------------------------------------------

function x = thresh(x, th, val)

[row col] = size(x);
for i=1:row
    for j=1:col
        if x(i,j) >= th(1) && x(i, j) <= th(2)
            x(i, j) = val;
        else
            x(i, j) = 0;
        end
    end
end

return;

%--------------------------------------------------------------------------

== matlab function  Blob Detection and Tracking (Enabled)/find blobs ==
  data: BIN input double; r output double; g output double; b output double; n output double; type input double
function [r, g, b, n]  = find_blobs(BIN, type)
% This block supports the Embedded MATLAB subset.
% See the help menu for details. 

idvec = zeros(1, 50);

[ROW COL] = size(BIN);

%{
if ROW>120 || COL>160
    r = uint8(BIN);
    g = uint8(BIN);
    b = uint8(BIN);
    n = -1;
    return;
end
%}

dwnsmple = 4;
row = round(ROW/dwnsmple);
col = round(COL/dwnsmple);
bin = uint8(zeros(row, col));

rw = 0;
% for i=dwnsmple+1:dwnsmple:ROW
for i=1:dwnsmple:ROW
    rw = rw + 1;
    co = 0;
    for j=1:dwnsmple:COL
        co = co + 1;
        bin(rw, co) = uint8(BIN(i, j));
    end
end

% r = uint8(zeros(row, col));
% g = uint8(zeros(row, col));
% b = uint8(zeros(row, col));
r = uint8(bin);
g = uint8(bin);
b = uint8(bin);
n = -1;%count;

% Bin = double(bin)/255;
% binsum = sum(Bin(:));
% ratio = binsum/(row*col);

% if ratio<=0.1
    % Find the 4 or 8 connected reachability matrix
    [eqtable, limg, maxlabel] = find_reachability_matrix(bin, type);
    if maxlabel>=1
        % Find equivalent labels
        table1 = updatetable(eqtable, maxlabel);
        table2 = updatetable2(table1, maxlabel);
        table3 = double(or(table1, table2));
        [idvec, n] = updatetable3(table3, maxlabel);
%     
%     
%         % Label the final image
        Limg = label_image(limg, n, idvec, maxlabel);
        r = uint8(Limg);
        g = uint8(Limg);
        b = uint8(Limg);
    end
%     r = uint8(limg);
%     g = uint8(limg);
%     b = uint8(limg);
% end



return;
%--------------------------------------------------------------------------
function [eqtable, limg, maxlabel] = find_reachability_matrix(img, Type)

[row col] = size(img);

type = Type;
if Type~=4 && Type~=8
    type = 8;
end

% Step 1: Label 8 or 4 connected components
limg = zeros(row, col);
label = 0;
Maxlabel = 50;
for i=1:row
    for j=1:col
        if img(i, j)>0 && limg(i, j)==0
            if (j-1)>=1 && img(i, j-1)>0
                limg(i, j)= limg(i, j-1);
            else
                if label<=(Maxlabel-1)
                    label = label+1;
                    limg(i, j)= label;
                else
                    limg(i, j)= 0;
                end
            end
        end
    end
end

% Find the reachability matrix
maxlabel = label;
eqtable = eye(Maxlabel, Maxlabel);
if maxlabel<1
    return;
end
% eqtable = eye(maxlabel, maxlabel);
for i=2:row
    for j=1:col
        if type == 4
            if img(i, j)>0
                if img(i-1, j)>0 && limg(i, j)~=0
                    eqtable(limg(i, j), limg(i-1, j)) = 1;
                    eqtable(limg(i-1, j), limg(i, j)) = 1;
                end
            end
        elseif type == 8
            if img(i, j)>0 && limg(i, j)~=0
                if (j-1)>=1 && img(i-1, j-1)>0 
                    eqtable(limg(i, j), limg(i-1, j-1)) = 1;
                    eqtable(limg(i-1, j-1), limg(i, j)) = 1;
                end
                if img(i-1, j)>0
                    eqtable(limg(i, j), limg(i-1, j)) = 1;
                    eqtable(limg(i-1, j), limg(i, j)) = 1;
                end
                if (j+1)<=col && img(i-1, j+1)>0
                    eqtable(limg(i, j), limg(i-1, j+1)) = 1;
                    eqtable(limg(i-1, j+1), limg(i, j)) = 1;
                end
            end
        end
        
    end
end

return;
%--------------------------------------------------------------------------
function [table] = updatetable(eqtable, maxlabel)

[row col] = size(eqtable);
table = zeros(row, col);
% etable = eqtable;
for i=1:maxlabel
    tmp1 = eqtable(i, :);
    for j=i+1:maxlabel
        tmp2 = eqtable(j, :);
        iscommon = sum(double(and(tmp1, tmp2)));
        if iscommon
            tmp1 = double(or(tmp1, tmp2));
        end
    end
        table(i, :) = tmp1;
end

return;
%--------------------------------------------------------------------------
function [table] = updatetable2(eqtable, maxlabel)

[row col] = size(eqtable);
table = zeros(row, col);
% etable = eqtable;
for i=maxlabel:-1:1
    tmp1 = eqtable(i, :);
%         i
%         count = count + 1;
%         idvec(i) = count;
    for j=i-1:-1:1
        tmp2 = eqtable(j, :);
        iscommon = sum(double(and(tmp1, tmp2)));
        if iscommon
            tmp1 = double(or(tmp1, tmp2));
%                 find(tmp1==1)
%                 pause
        end
    end
    table(i, :) = tmp1;
end

return;
%--------------------------------------------------------------------------
function [idvec, count] = updatetable3(eqtable, maxlabel)

[row col] = size(eqtable);
table = zeros(row, col);
count = 0;
idvec = zeros(1, col);
% etable = eqtable;
for i=1:maxlabel
    tmp1 = eqtable(i, :);
    if tmp1(i)~=0
        count = count + 1;
        idvec(i) = count;
        for j=i+1:maxlabel
            tmp2 = eqtable(j, :);
            iscommon = sum(double(and(tmp1, tmp2)));
            if iscommon
                tmp1 = double(or(tmp1, tmp2));
            end
        end
        table(i, :) = tmp1;
        for j=i+1:maxlabel
            if tmp1(j)==1
                idvec(j) = count;
                eqtable(j, :) = table(j, :);
            end
        end
    end
end

return;
%--------------------------------------------------------------------------
function [Limg] = label_image(limg, count, idvec, maxlabel)

[row col] = size(limg);
Limg = limg;
for i=1:row
    for j=1:col
        if Limg(i, j)>0 && Limg(i, j)<=maxlabel
%             if count<=255
%                 Limg(i, j) = uint8(round((255/count)*idvec(Limg(i, j))));
%             else
                Limg(i, j) = uint8(idvec(Limg(i, j)));
%             end
        end
    end
end

return;
%--------------------------------------------------------------------------

== matlab function QBot 2e Ful _Kinematics (No Gyro)/Qbot2e_Kinematics (No Gyro)/Qbot2_Kinematics (Vf,W to x_dot,y_dot and psi_dot) ==
  data: vC input double; x_dot output double; Omega input double; y_dot output double; psi input double; psi_dot output double
function [x_dot,y_dot,psi_dot] = fcn(vC,Omega,psi)
%#codegen


x_dot=cos(psi)*vC;
y_dot=sin(psi)*vC;
psi_dot= Omega;

== matlab function QBot 2e Inverse Kinematics (Forward Velocity and Angular Velocity into Left and Right Wheel Vellocity)/QBot2e_Inverse_Kinematics (Forward Velocity and Angular Velocity into Left and Right Wheel Vellocity) ==
  data: vR output double; vL output double; vC input double; Omega input double
function [vR,vL] = fcn(vC , Omega)
%#codegen

d=0.235; 
% Eqn Based on the eqn 4.52 (W is the angular velocity)

vR = vC + Omega*d/2;
vL= vC - Omega*d/2;
